simulink model "Navigation_Sim"  (R2023b)
settings: Solver=FixedStepAuto  StartTime=0.0  StopTime=tf  FixedStep=tstep  RelTol=1e-3
values from neighbouring files (symbols this model uses):
  Ixx = 1    [Navigation_Script.m]
  Iyy = 1.1    [Navigation_Script.m]
  Izz = 0.9    [Navigation_Script.m]
  L = 0.01    [Navigation_Script.m]
  M = 0.02    [Navigation_Script.m]
  N = -0.03    [Navigation_Script.m]
  P0 = zeros(4,4)    [Navigation_Script.m]
  Q = 0.000001.*eye(4)    [Navigation_Script.m]
  R = 1.*eye(4)    [Navigation_Script.m]
  tstep = 0.001    [Navigation_Script.m]
libraries: simulink x2
settings Model: Creator=1537565965A  LastModifiedBy=Nathan Dablain
settings SolverCC: AlgebraicLoopSolver=TrustRegion
settings DebuggingCC: UnconnectedInputMsg=warning  UnconnectedOutputMsg=warning  UnconnectedLineMsg=warning
settings ModelReferenceCC: EnableRefExpFcnMdlSchedulingChecks=on
settings SFSimCC: CustomCodeUndefinedFunction=UseInterfaceOnly

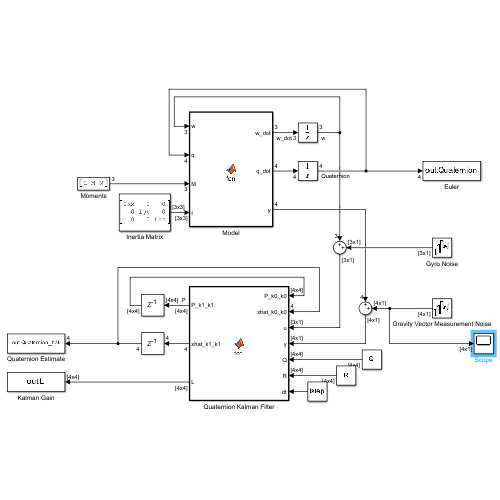
[thumbnail: Simulink's stored preview of the top-level diagram]
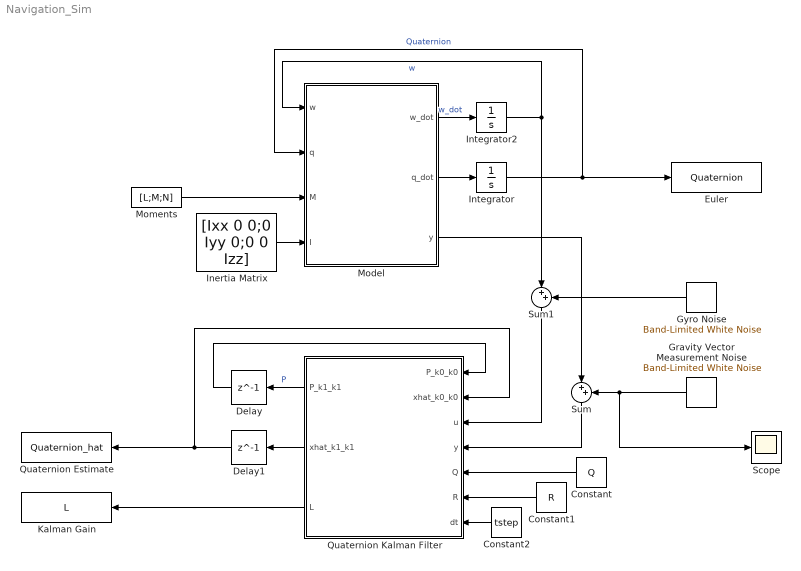
== system Navigation_Sim ==
  Constant : Constant  Value=Q
  Constant1 : Constant  Value=R
  Constant2 : Constant  Value=tstep
  Delay : Delay  DelayLength=1  InitialCondition=P0
  Delay1 : Delay  DelayLength=1  InitialCondition=[1;0;0;0]
  Euler : ToWorkspace  VariableName=Quaternion  SaveFormat=Structure  SampleTime=-1
  Gravity Vector Measurement Noise : simulink/Sources/Band-Limited White Noise  Cov=[1; 1; 1; 1].*(tstep^2)  Ts=tstep  seed=[23341]  VectorParams1D=off
  Gyro Noise : simulink/Sources/Band-Limited White Noise  Cov=[1; 1; 1].*tstep^2  Ts=tstep  seed=[23341]  VectorParams1D=off
  Inertia Matrix : Constant  Value=[Ixx 0 0;0 Iyy 0;0 0 Izz]
  Integrator : Integrator  InitialCondition=[1;0;0;0]
  Integrator2 : Integrator  InitialCondition=zeros(3,1)
  Kalman Gain : ToWorkspace  VariableName=L  SaveFormat=Structure  SampleTime=-1
  Model : MATLAB Function  TreatAsAtomicUnit=on
  Moments : Constant  Value=[L;M;N]
  Quaternion Estimate : ToWorkspace  VariableName=Quaternion_hat  SaveFormat=Structure  SampleTime=-1
  Quaternion Kalman Filter : MATLAB Function  TreatAsAtomicUnit=on
  Scope : Scope
  Sum : Sum  Inputs=|++
  Sum1 : Sum  Inputs=|++
  wires:
  Integrator/1 -> Euler/1, Model/2(q)  "Quaternion"
  Model/1(w_dot) -> Integrator2/1  "w_dot"
  Integrator2/1 -> Sum1/1, Model/1(w)  "w"
  Inertia Matrix/1 -> Model/4(I)
  Model/2(q_dot) -> Integrator/1
  Quaternion Kalman Filter/1(P_k1_k1) -> Delay/1  "P"
  Quaternion Kalman Filter/2(xhat_k1_k1) -> Delay1/1
  Delay/1 -> Quaternion Kalman Filter/1(P_k0_k0)
  Delay1/1 -> Quaternion Kalman Filter/2(xhat_k0_k0), Quaternion Estimate/1
  Gravity Vector Measurement Noise/1 -> Scope/1, Sum/2
  Sum/1 -> Quaternion Kalman Filter/4(y)
  Constant/1 -> Quaternion Kalman Filter/5(Q)
  Constant1/1 -> Quaternion Kalman Filter/6(R)
  Constant2/1 -> Quaternion Kalman Filter/7(dt)
  Gyro Noise/1 -> Sum1/2
  Sum1/1 -> Quaternion Kalman Filter/3(u)
  Quaternion Kalman Filter/3(L) -> Kalman Gain/1
  Moments/1 -> Model/3(M)
  Model/3(y) -> Sum/1

== matlab function Navigation_Sim/Quaternion Kalman Filter ==
  data: P_k0_k0 input; xhat_k0_k0 input; u input; P_k1_k1 output; y input; xhat_k1_k1 output; Q input; R input; dt input; L output
function [P_k1_k1,xhat_k1_k1,L] = fcn(P_k0_k0,xhat_k0_k0,u,y,Q,R,dt)
wx = u(1);
wy = u(2);
wz = u(3);
q0 = xhat_k0_k0(1);
q1 = xhat_k0_k0(2);
q2 = xhat_k0_k0(3);
q3 = xhat_k0_k0(4);
g = 9.81;

% c2 = 2*q0*q1*dt;
% c3 = 2*q0*q2*dt;
% c4 = 2*q0*q3*dt;
% c5 = 2*q1*q2*dt;
% c6 = 2*q1*q3*dt;
% c7 = 2*q2*q3*dt;

c8 = (dt*wx)/2;
c9 = (dt*wy)/2;
c10 = (dt*wz)/2;

H = 2*g.*[q0/g q1/g q2/g q3/g;...
          q2 q3 q0 q1;...
          -q1 -q0 q3 q2;...
          q0 -q1 -q2 q3];
% F = [1-(3*q0^2)+dt c8-c2 c9-c3 c10-c4;...
%      -c8-c2 1-(3*q1^2)+dt c10-c5 -c9-c6;...
%      -c9-c3 -c10-c5 1-(3*q2^2)+dt c8-c7;...
%      -c10-c4 c9-c6 -c8-c7 1-(3*q3^2)+dt];
F = [1 c8 c9 c10;...
     -c8 1 c10 -c9;...
     -c9 -c10 1 c8;...
     -c10 c9 -c8 1];
xhat_k1_k0 = xhat_k0_k0 + dt.*[(q1*wx)/2 + (q2*wy)/2 + (q3*wz)/2 - q0*(q0^2 + q1^2 + q2^2 + q3^2 - 1);...
                               -1*((q0*wx)/2 + (q3*wy)/2 - (q2*wz)/2 + q1*(q0^2 + q1^2 + q2^2 + q3^2 - 1));...
                               -1*((q0*wy)/2 - (q3*wx)/2 + (q1*wz)/2 + q2*(q0^2 + q1^2 + q2^2 + q3^2 - 1));...
                               -1*((q2*wx)/2 - (q1*wy)/2 + (q0*wz)/2 + q3*(q0^2 + q1^2 + q2^2 + q3^2 - 1))];
yhat = [xhat_k1_k0(1)^2+xhat_k1_k0(2)^2+xhat_k1_k0(3)^2+xhat_k1_k0(4)^2;...
        2*g*xhat_k1_k0(1)*xhat_k1_k0(3) + 2*g*xhat_k1_k0(2)*xhat_k1_k0(4);...
        2*g*xhat_k1_k0(3)*xhat_k1_k0(4) - 2*g*xhat_k1_k0(1)*xhat_k1_k0(2);...
        g*(xhat_k1_k0(1)^2-xhat_k1_k0(2)^2-xhat_k1_k0(3)^2+xhat_k1_k0(4)^2)];
P_k1_k0 = F*P_k0_k0*F' + Q;
ybar = y-yhat;
S = H*P_k1_k0*H' + R;
L = P_k1_k0*H'*inv(S);
xhat_k1_k1 = xhat_k1_k0 + L*ybar;
P_k1_k1 = (eye(4)-L*H)*P_k1_k0;
end

== matlab function Navigation_Sim/Model ==
  data: w input; q input; w_dot output; M input; I input; q_dot output; y output
function [w_dot,q_dot,y] = fcn(w,q,M,I)
    g = 9.81;
    w_dot = I\(M-cross(w,I*w));
    omega = 0.5.*[0      w(1)    w(2)    w(3);...
             -w(1)  0       w(3)     -w(2);...
             -w(2)  -w(3)   0       w(1);...
             -w(3)  w(2)    -w(1)   0];
    q_dot = (omega*q)+((1-dot(q,q))*q);
    y = [0;...
        2*g*q(1)*q(3) + 2*g*q(2)*q(4);...
        2*g*q(3)*q(4) - 2*g*q(1)*q(2);...
        g*q(1)^2 - g*q(2)^2 - g*q(3)^2 + g*q(4)^2];
end
